simulink model "acc_test"  (R2018b)
settings: Solver=VariableStepAuto  StartTime=0.0  StopTime=20  RelTol=1e-3
values from neighbouring files (symbols this model uses):
  g0 = 2    [acc_sim_parameters.m]
  Ks = 2    [acc_sim_parameters.m]
  Kv = 1    [acc_sim_parameters.m]
  lr = 1.6    [acc_sim_parameters.m]    (also in lat_sim_parameters.m = 2; tuneLateralController.m = 2)
  m = 1575    [acc_sim_parameters.m]    (also in lat_sim_parameters.m = 2000; tuneLateralController.m = 2000)
  maxAcc = 3    [acc_sim_parameters.m]
  minAcc = -3    [acc_sim_parameters.m]
  tau = 0.5    [acc_sim_parameters.m]
  timeGap = 1    [acc_sim_parameters.m]
libraries: autolibshared x2
settings Model: Creator=Fernando VM  LastModifiedBy=Fernando VM

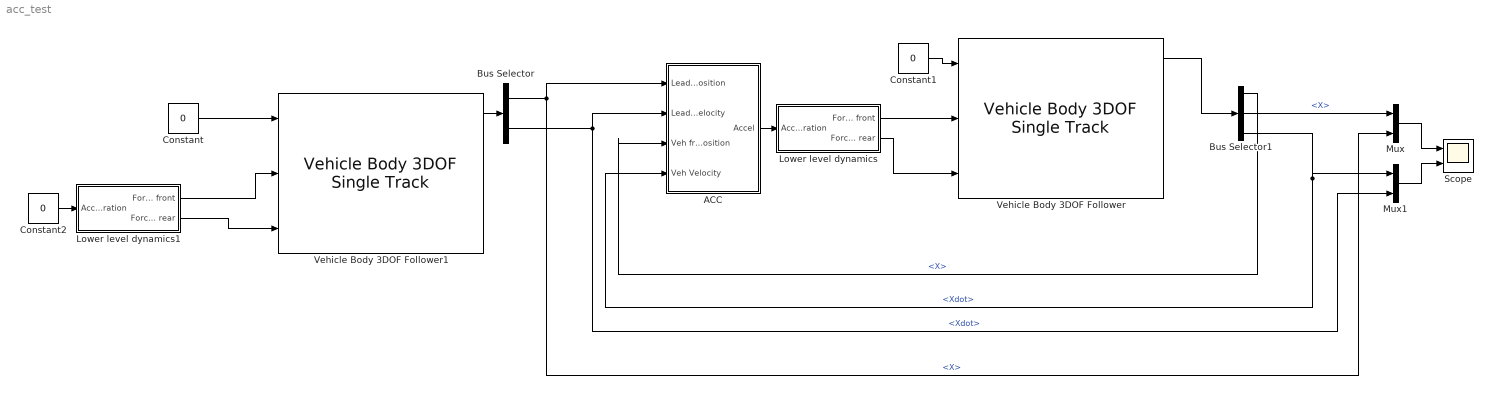
== system acc_test ==
  ACC : Subsystem
  Bus Selector : BusSelector  OutputSignals=InertFrm.RearAxl.Disp.X,InertFrm.RearAxl.Vel.Xdot
  Bus Selector1 : BusSelector  OutputSignals=InertFrm.FrntAxl.Disp.X,InertFrm.RearAxl.Disp.X,InertFrm.RearAxl.Vel.Xdot
  Constant : Constant  Value=0
  Constant1 : Constant  Value=0
  Constant2 : Constant  Value=0
  Lower level dynamics : Subsystem
  Lower level dynamics1 : Subsystem
  Mux : Mux  Inputs=2
  Mux1 : Mux  Inputs=2
  Scope : Scope  NumInputPorts=2
  Vehicle Body 3DOF Follower : autolibshared/Vehicle Body 3DOF Single Track  trackMode=Single (bicycle)  inputMode=External longitudinal forces  frontSteerMode=on  rearSteerMode=off  windMode=off  muMode=off  extFMode=off  extMMode=off  aMode=2  NF=2  NR=2  m=m  a=lf  b=lr  h=0.35  X_o=follInitPos  xdot_o=follInitVel  CalphaMode=off  sigmaMode=on  d=0  w=[1.4,1.4]  Cy_f=Cf  Cy_r=Cr  sigma_f=.1  sigma_r=.1  alpha_f_brk=[-.1 .1]  Cy_f_data=[-9e3 9e3]  alpha_r_brk=[-.1 .1]  Cy_r_data=[-9e3 9e3]  Y_o=0  ydot_o=0  Izz=Iz  psi_o=0  r_o=0  Af=2  Cd=.3  Cl=.1  Cpm=.1  beta_w=[0:0.01:0.3]  Cs=[0:0.03:0.9]  Cym=[0:0.01:0.3]  Pabs=101325  Tair=273  g=9.81  mu=1  xdot_tol=.01  Fznom=5000  Fxtire_sat=7e4  Fytire_sat=7e4  longOff=0  latOff=0  vertOff=0
      settings: SourceProductName=Powertrain Blockset  SourceProductBaseCode=PW
  Vehicle Body 3DOF Follower1 : autolibshared/Vehicle Body 3DOF Single Track  trackMode=Single (bicycle)  inputMode=External longitudinal forces  frontSteerMode=on  rearSteerMode=off  windMode=off  muMode=off  extFMode=off  extMMode=off  aMode=2  NF=2  NR=2  m=m  a=lf  b=lr  h=0.35  X_o=leaderInitPos  xdot_o=leaderInitVel  CalphaMode=off  sigmaMode=on  d=0  w=[1.4,1.4]  Cy_f=Cf  Cy_r=Cr  sigma_f=.1  sigma_r=.1  alpha_f_brk=[-.1 .1]  Cy_f_data=[-9e3 9e3]  alpha_r_brk=[-.1 .1]  Cy_r_data=[-9e3 9e3]  Y_o=0  ydot_o=0  Izz=Iz  psi_o=0  r_o=0  Af=2  Cd=.3  Cl=.1  Cpm=.1  beta_w=[0:0.01:0.3]  Cs=[0:0.03:0.9]  Cym=[0:0.01:0.3]  Pabs=101325  Tair=273  g=9.81  mu=1  xdot_tol=.01  Fznom=5000  Fxtire_sat=7e4  Fytire_sat=7e4  longOff=0  latOff=0  vertOff=0
      settings: SourceProductName=Powertrain Blockset  SourceProductBaseCode=PW
  wires:
  Constant/1 -> Vehicle Body 3DOF Follower1/1
  Constant1/1 -> Vehicle Body 3DOF Follower/1
  Constant2/1 -> Lower level dynamics1/1(Acceleration)
  Vehicle Body 3DOF Follower1/1 -> Bus Selector/1
  Vehicle Body 3DOF Follower/1 -> Bus Selector1/1
  Bus Selector1/3 -> ACC/4(Veh Velocity), Mux1/1  "<Xdot>"
  Bus Selector/1 -> ACC/1(Leader rear position), Mux/2  "<X>"
  Bus Selector/2 -> ACC/2(Leader Velocity), Mux1/2  "<Xdot>"
  Bus Selector1/2 -> Mux/1  "<X>"
  Mux/1 -> Scope/1
  Mux1/1 -> Scope/2
  Lower level dynamics/1(Forces front) -> Vehicle Body 3DOF Follower/2
  Lower level dynamics/2(Forces rear) -> Vehicle Body 3DOF Follower/3
  Lower level dynamics1/1(Forces front) -> Vehicle Body 3DOF Follower1/2
  Lower level dynamics1/2(Forces rear) -> Vehicle Body 3DOF Follower1/3
  ACC/1(Accel) -> Lower level dynamics/1(Acceleration)
  Bus Selector1/1 -> ACC/3(Veh front position)  "<X>"

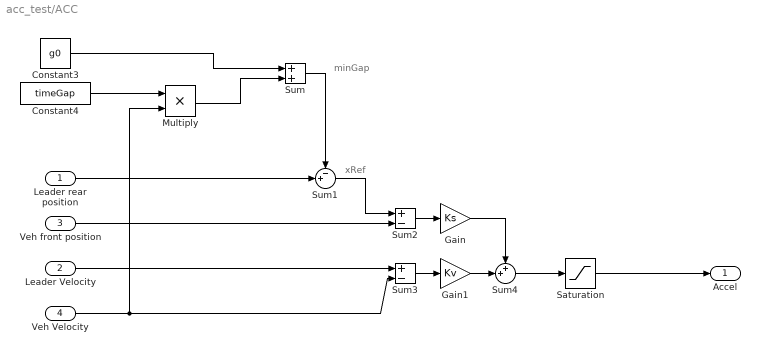
== system acc_test/ACC ==
  note: minGap
  note: xRef
  Leader rear position : Inport
  Leader Velocity : Inport  Port=2
  Veh front position : Inport  Port=3
  Veh Velocity : Inport  Port=4
  Constant3 : Constant  Value=g0
  Constant4 : Constant  Value=timeGap
  Gain : Gain  Gain=Ks
  Gain1 : Gain  Gain=Kv
  Multiply : Product
  Saturation : Saturate  UpperLimit=maxAcc  LowerLimit=minAcc
  Sum : Sum
  Sum1 : Sum  Inputs=-+|
  Sum2 : Sum  Inputs=+-
  Sum3 : Sum  Inputs=+-
  Sum4 : Sum  Inputs=++|
  Accel : Outport
  wires:
  Sum/1 -> Sum1/1
  Gain1/1 -> Sum4/2
  Sum3/1 -> Gain1/1
  Constant4/1 -> Multiply/1
  Multiply/1 -> Sum/2
  Leader rear position/1 -> Sum1/2
  Sum2/1 -> Gain/1
  Gain/1 -> Sum4/1
  Constant3/1 -> Sum/1
  Sum4/1 -> Saturation/1
  Veh Velocity/1 -> Sum3/2, Multiply/2
  Leader Velocity/1 -> Sum3/1
  Veh front position/1 -> Sum2/2
  Sum1/1 -> Sum2/1
  Saturation/1 -> Accel/1

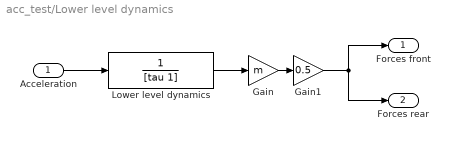
== system acc_test/Lower level dynamics ==
  Acceleration : Inport
  Gain : Gain  Gain=m
  Gain1 : Gain  Gain=0.5
  Lower level dynamics : TransferFcn  Denominator=[tau 1]
  Forces front : Outport
  Forces rear : Outport  Port=2
  wires:
  Gain/1 -> Gain1/1
  Gain1/1 -> Forces front/1, Forces rear/1
  Acceleration/1 -> Lower level dynamics/1
  Lower level dynamics/1 -> Gain/1

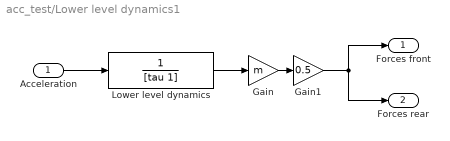
== system acc_test/Lower level dynamics1 ==
  Acceleration : Inport
  Gain : Gain  Gain=m
  Gain1 : Gain  Gain=0.5
  Lower level dynamics : TransferFcn  Denominator=[tau 1]
  Forces front : Outport
  Forces rear : Outport  Port=2
  wires:
  Gain/1 -> Gain1/1
  Gain1/1 -> Forces front/1, Forces rear/1
  Acceleration/1 -> Lower level dynamics/1
  Lower level dynamics/1 -> Gain/1
